simulink model "Sedackaa"  (R2022b)
settings: Solver=VariableStepAuto  StartTime=0.0  StopTime=5  RelTol=1e-3
settings Model: Creator=honza  LastModifiedBy=honza

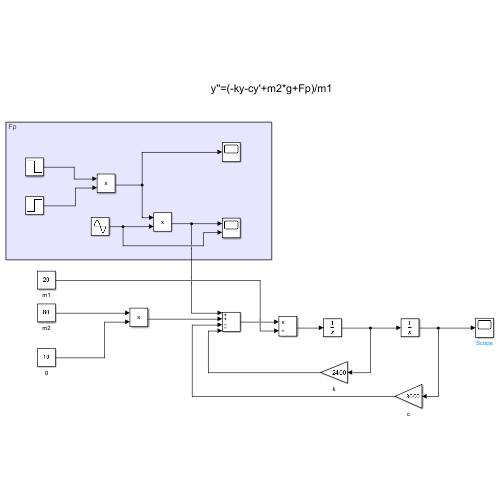
[thumbnail: Simulink's stored preview of the top-level diagram]
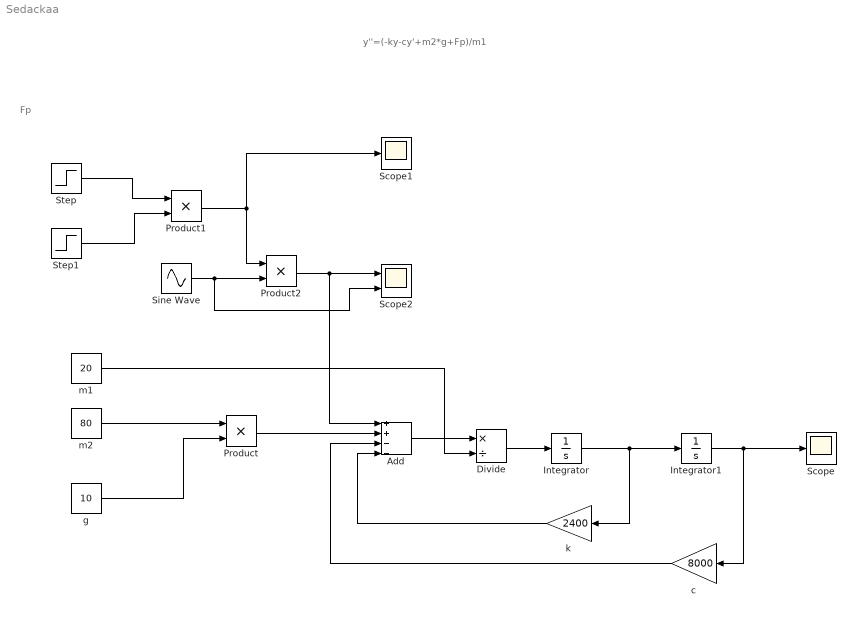
== system Sedackaa ==
  note: y''=(-ky-cy'+m2*g+Fp)/m1
  note: Fp
  Add : Sum  Inputs=++--
  Divide : Product  Inputs=*/
  Integrator : Integrator
  Integrator1 : Integrator
  Product : Product
  Product1 : Product
  Product2 : Product
  Scope : Scope
  Scope1 : Scope
  Scope2 : Scope  NumInputPorts=2
  Sine Wave : Sin  Amplitude=-0.2*10*80  Frequency=2*pi  Phase=pi  SampleTime=0
  Step : Step  Time=2  Before=1  After=0  SampleTime=0
  Step1 : Step  Time=1.5  SampleTime=0
  c : Gain  Gain=8000
  g : Constant  Value=10
  k : Gain  Gain=2400
  m1 : Constant  Value=20
  m2 : Constant  Value=80
  wires:
  Integrator/1 -> k/1, Integrator1/1
  Integrator1/1 -> Scope/1, c/1
  Add/1 -> Divide/1
  Divide/1 -> Integrator/1
  m1/1 -> Divide/2
  m2/1 -> Product/1
  g/1 -> Product/2
  Step/1 -> Product1/1
  Step1/1 -> Product1/2
  Product1/1 -> Scope1/1, Product2/1
  Sine Wave/1 -> Scope2/2, Product2/2
  Product2/1 -> Add/1, Scope2/1
  Product/1 -> Add/2
  k/1 -> Add/4
  c/1 -> Add/3
